simulink model "chap04"  (R2021a)
settings: Solver=FixedStepDiscrete  StartTime=0.0  StopTime=30  FixedStep=0.001  RelTol=1e-3
undefined symbols (not defined in the file): DiscIntNeverNeededParam
libraries: simulink x4
(part 1 of 7)
settings Model: Creator=陈天兴  LastModifiedBy=陈天兴

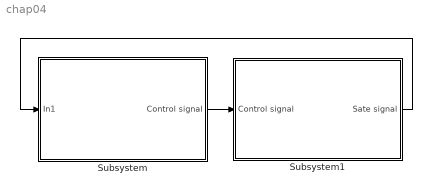
== system chap04 ==
  Subsystem : Subsystem
  Subsystem1 : Subsystem
  wires:
  Subsystem/1(Control signal) -> Subsystem1/1(Control signal)
  Subsystem1/1(Sate signal) -> Subsystem/1(In1)

== system chap04/Subsystem ==
  In1 : Inport
  Bus Creator : BusCreator  Inputs=6
  Bus Creator1 : BusCreator  Inputs=6
  Bus Creator2 : BusCreator  Inputs=3
  Subsystem : Subsystem
  Subsystem1 : Subsystem
  Subsystem10 : Subsystem
  Subsystem11 : Subsystem
  Subsystem13 : Subsystem
  Subsystem2 : Subsystem
  Subsystem3 : Subsystem
  Subsystem4 : Subsystem
  Subsystem5 : Subsystem
  Subsystem6 : Subsystem
  Subsystem7 : Subsystem
  Subsystem9 : Subsystem
  Control signal : Outport
  wires:
  Bus Creator2/1 -> Subsystem13/1(In19), Subsystem9/1(In19), Subsystem7/1(In19), Subsystem11/1(In19), Subsystem10/1(In19), Subsystem6/1(In19), Subsystem/1(In19), Subsystem2/1(In19), Subsystem5/1(In19), Subsystem4/1(In19), Subsystem1/1(In19), Subsystem3/1(In19)
  Subsystem5/1(u3) -> Bus Creator/3
  Subsystem3/1(u4) -> Bus Creator/4
  Subsystem1/1(u5) -> Bus Creator/5
  Subsystem/1(u1) -> Bus Creator/1
  Subsystem2/1(u2) -> Bus Creator/2
  Subsystem4/1(u6) -> Bus Creator/6
  Bus Creator/1 -> [control], Control signal/1
  Subsystem10/1(u4) -> Bus Creator1/4
  In1/1 -> Bus Creator2/2  "state(t)"
  Bus Creator1/1 -> Bus Creator2/1  "state(tk)"
  Subsystem6/1(u1) -> Bus Creator1/1
  Subsystem13/1(u2) -> Bus Creator1/2
  Subsystem9/1(u3) -> Bus Creator1/3
  Subsystem7/1(u5) -> Bus Creator1/5
  Subsystem11/1(u6) -> Bus Creator1/6
  [control] -> Bus Creator2/3  "control"

== system chap04/Subsystem1 ==
  Control signal : Inport
  Bus Creator : BusCreator  Inputs=7
  Bus Creator1 : BusCreator  Inputs=6
  Bus Selector : BusSelector  OutputSignals=node1.ux,node1.uy,node1.uz
  Bus Selector1 : BusSelector  OutputSignals=node2.ux,node2.uy,node2.uz
  Bus Selector2 : BusSelector  OutputSignals=node3.ux,node3.uy,node3.uz
  Bus Selector3 : BusSelector  OutputSignals=node4.ux,node4.uy,node4.uz
  Bus Selector4 : BusSelector  OutputSignals=node5.ux,node5.uy,node5.uz
  Bus Selector5 : BusSelector  OutputSignals=node6.ux,node6.uy,node6.uz
  Constant2 : Constant
  Scope : Scope  NumInputPorts=3
  Subsystem : Subsystem
  Subsystem1 : Subsystem
  Subsystem2 : Subsystem
  Subsystem3 : Subsystem
  Subsystem4 : Subsystem
  Subsystem5 : Subsystem
  Subsystem6 : Subsystem
  Subsystem7 : Subsystem
  Sate signal : Outport
  wires:
  Bus Creator/1 -> Sate signal/1
  Control signal/1 -> Bus Selector/1, Bus Selector1/1, Bus Selector5/1, Bus Selector4/1, Bus Selector3/1, Bus Selector2/1
  Bus Selector/1 -> Subsystem/4(ut1x)  "<ux>"
  Bus Selector/2 -> Subsystem/5(ut1y)  "<uy>"
  Bus Selector/3 -> Subsystem/6(ut1z)  "<uz>"
  Bus Selector1/1 -> Subsystem1/4(ut2x)  "<ux>"
  Bus Selector1/2 -> Subsystem1/5(ut2y)  "<uy>"
  Bus Selector1/3 -> Subsystem1/6(ut2z)  "<uz>"
  Bus Selector2/1 -> Subsystem2/4(ut3x)  "<ux>"
  Bus Selector2/2 -> Subsystem2/5(ut3y)  "<uy>"
  Bus Selector2/3 -> Subsystem2/6(ut3z)  "<uz>"
  Bus Selector3/1 -> Subsystem3/4(ut4x)  "<ux>"
  Bus Selector3/2 -> Subsystem3/5(ut4y)  "<uy>"
  Bus Selector3/3 -> Subsystem3/6(ut4z)  "<uz>"
  Bus Selector4/1 -> Subsystem4/4(ut5x)  "<ux>"
  Bus Selector4/2 -> Subsystem4/5(ut5y)  "<uy>"
  Bus Selector4/3 -> Subsystem4/6(ut5z)  "<uz>"
  Bus Selector5/1 -> Subsystem5/4(ut6x)  "<ux>"
  Bus Selector5/2 -> Subsystem5/5(ut6y)  "<uy>"
  Bus Selector5/3 -> Subsystem5/6(ut6z)  "<uz>"
  Subsystem5/1(node6) -> Bus Creator/7
  Subsystem4/1(node5) -> Bus Creator/6
  Subsystem3/1(node4) -> Bus Creator/5
  Subsystem2/1(node3) -> Bus Creator/4
  Subsystem1/1(node2) -> Bus Creator/3
  Subsystem/1(node1) -> Bus Creator/2
  Subsystem6/5(vy) -> Bus Creator1/5  "vy"
  Subsystem6/2(xy) -> Bus Creator1/2  "xy"
  Subsystem6/3(xz) -> Bus Creator1/3  "xz"
  Subsystem6/4(vx) -> Bus Creator1/4  "vx"
  Subsystem6/6(vz) -> Bus Creator1/6  "vz"
  Bus Creator1/1 -> Bus Creator/1  "node0"
  Subsystem6/1(xx) -> Bus Creator1/1  "xx"
  Subsystem7/2(dy) -> Subsystem/2(dy), Subsystem5/2(dy), Subsystem4/2(dy), Subsystem3/2(dy), Subsystem2/2(dy), Subsystem1/2(dy), Scope/2  "dy"
  Subsystem7/3(dz) -> Subsystem5/3(dz), Subsystem4/3(dz), Subsystem3/3(dz), Subsystem2/3(dz), Subsystem1/3(dz), Subsystem/3(dz), Scope/3  "dz"
  Subsystem7/1(dx) -> Subsystem3/1(dx), Subsystem5/1(dx), Subsystem4/1(dx), Subsystem2/1(dx), Subsystem1/1(dx), Subsystem/1(dx), Scope/1  "dx"
  Constant2/1 -> Subsystem7/1(switch)

== system chap04/Subsystem/Subsystem ==
  In19 : Inport
  Bus Creator : BusCreator  Inputs=3
  Bus Selector : BusSelector  OutputSignals=state(tk).node1.xx,state(tk).node2.xx,state(tk).node3.xx,state(tk).node6.xx,state(tk).node1.vx,state(tk).node2.vx,state(tk).node3.vx,state(tk).node6.vx
  Bus Selector1 : BusSelector  OutputSignals=state(tk).node1.xy,state(tk).node2.xy,state(tk).node3.xy,state(tk).node6.xy,state(tk).node1.vy,state(tk).node2.vy,state(tk).node3.vy,state(tk).node6.vy
  Bus Selector2 : BusSelector  OutputSignals=state(tk).node1.xz,state(tk).node2.xz,state(tk).node3.xz,state(tk).node6.xz,state(tk).node1.vz,state(tk).node2.vz,state(tk).node3.vz,state(tk).node6.vz
  Bus Selector3 : BusSelector  OutputSignals=state(t).node1.vx
  Bus Selector4 : BusSelector  OutputSignals=state(t).node1.vy
  Bus Selector5 : BusSelector  OutputSignals=state(t).node1.vz
  Bus Selector6 : BusSelector  OutputSignals=state(t).node1.vx,state(t).node1.vy,state(t).node1.vz
  Bus Selector7 : BusSelector  OutputSignals=state(t).node1.vx,state(t).node1.vy,state(t).node1.vz
  Bus Selector8 : BusSelector  OutputSignals=control.node1.ux,control.node1.uy,control.node1.uz
  Subsystem1 : Subsystem
  Subsystem10 : Subsystem
  Subsystem12 : Subsystem
  Subsystem2 : Subsystem
  Subsystem3 : Subsystem
  Subsystem4 : Subsystem
      settings: PortSchema="{\"entries\":[{\"content\":{\"sides\":[{\"content\":{\"connectorIds\":[\"In1\",\"In2\",\"In3\"]},\"type\":\"ConnectorPlacement.EquallySpacedRectSide\",\"uuid\":\"3c32f130-2df4-4697-80e9-267a8217898e\"},{\"content\":{\"connectorIds\":[\"Out1\"],\"side\":\"RIGHT\"},\"type\":\"ConnectorPlacement.EquallySpacedRectSide\",\"uuid\":\"840675a7-4714-440f-a6ce-75eff1b2763f\"},{\"content\":{\"connectorIds\":[],\"side\":\"TOP\"},\"type\":\"ConnectorPlacement.EquallySpacedRectSide\",\"uuid\":\"5c23af56-4ec3-4a39-a531-12998a0be3c8\"},{\"content\":{\"connectorIds\":[\"Out2\"],\"side\":\"BOTTOM\"},\"type\":\"ConnectorPlacement.EquallySpacedRectSide\",\"uuid\":\"31d953fb-65a0-42e9-a844-060de010f298\"}]},\"type\":\"ConnectorPlacement.EquallySpacedConnector\",\"uuid\":\"61b27aa3-5880-401e-bae3-4611093a191a\"}],\"packageUris\":[\"http://schema.mathworks.com/mf0/Connector/R2020b\"],\"version\":\"1.0\"}"
  Subsystem6 : Subsystem
  Subsystem7 : Subsystem
      settings: PortSchema="{\"entries\":[{\"content\":{\"sides\":[{\"content\":{\"connectorIds\":[\"In1\",\"In2\",\"In3\"]},\"type\":\"ConnectorPlacement.EquallySpacedRectSide\",\"uuid\":\"3c32f130-2df4-4697-80e9-267a8217898e\"},{\"content\":{\"connectorIds\":[\"Out1\"],\"side\":\"RIGHT\"},\"type\":\"ConnectorPlacement.EquallySpacedRectSide\",\"uuid\":\"840675a7-4714-440f-a6ce-75eff1b2763f\"},{\"content\":{\"connectorIds\":[],\"side\":\"TOP\"},\"type\":\"ConnectorPlacement.EquallySpacedRectSide\",\"uuid\":\"5c23af56-4ec3-4a39-a531-12998a0be3c8\"},{\"content\":{\"connectorIds\":[\"Out2\"],\"side\":\"BOTTOM\"},\"type\":\"ConnectorPlacement.EquallySpacedRectSide\",\"uuid\":\"31d953fb-65a0-42e9-a844-060de010f298\"}]},\"type\":\"ConnectorPlacement.EquallySpacedConnector\",\"uuid\":\"61b27aa3-5880-401e-bae3-4611093a191a\"}],\"packageUris\":[\"http://schema.mathworks.com/mf0/Connector/R2020b\"],\"version\":\"1.0\"}"
  Subsystem8 : Subsystem
      settings: PortSchema="{\"entries\":[{\"content\":{\"sides\":[{\"content\":{\"connectorIds\":[\"In1\",\"In2\",\"In3\"]},\"type\":\"ConnectorPlacement.EquallySpacedRectSide\",\"uuid\":\"3c32f130-2df4-4697-80e9-267a8217898e\"},{\"content\":{\"connectorIds\":[\"Out1\"],\"side\":\"RIGHT\"},\"type\":\"ConnectorPlacement.EquallySpacedRectSide\",\"uuid\":\"840675a7-4714-440f-a6ce-75eff1b2763f\"},{\"content\":{\"connectorIds\":[],\"side\":\"TOP\"},\"type\":\"ConnectorPlacement.EquallySpacedRectSide\",\"uuid\":\"5c23af56-4ec3-4a39-a531-12998a0be3c8\"},{\"content\":{\"connectorIds\":[\"Out2\"],\"side\":\"BOTTOM\"},\"type\":\"ConnectorPlacement.EquallySpacedRectSide\",\"uuid\":\"31d953fb-65a0-42e9-a844-060de010f298\"}]},\"type\":\"ConnectorPlacement.EquallySpacedConnector\",\"uuid\":\"61b27aa3-5880-401e-bae3-4611093a191a\"}],\"packageUris\":[\"http://schema.mathworks.com/mf0/Connector/R2020b\"],\"version\":\"1.0\"}"
  u1 : Outport
  wires:
  Subsystem2/1(utx) -> Subsystem8/2(utz)
  Subsystem6/1(utx) -> Subsystem4/2(utx)
  Subsystem1/1(utx) -> Subsystem7/2(uty)
  Bus Creator/1 -> u1/1  "node1"
  In19/1 -> [state], Bus Selector2/1, Bus Selector/1, Bus Selector1/1
  Bus Selector/1 -> Subsystem6/1(xx1)  "<xx>"
  Bus Selector/2 -> Subsystem6/2(xx2)  "<xx>"
  Bus Selector/3 -> Subsystem6/3(xx3)  "<xx>"
  Bus Selector/4 -> Subsystem6/4(xx6)  "<xx>"
  Bus Selector/5 -> Subsystem6/5(vx1)  "<vx>"
  Bus Selector/6 -> Subsystem6/6(vx2)  "<vx>"
  Bus Selector/7 -> Subsystem6/7(vx3)  "<vx>"
  Bus Selector/8 -> Subsystem6/8(vx6)  "<vx>"
  Bus Selector1/1 -> Subsystem1/1(xy1)  "<xy>"
  Bus Selector1/2 -> Subsystem1/2(xy2)  "<xy>"
  Bus Selector1/3 -> Subsystem1/3(xy3)  "<xy>"
  Bus Selector1/4 -> Subsystem1/4(xy6)  "<xy>"
  Bus Selector1/5 -> Subsystem1/5(vy1)  "<vy>"
  Bus Selector1/6 -> Subsystem1/6(vy2)  "<vy>"
  Bus Selector1/7 -> Subsystem1/7(vy3)  "<vy>"
  Bus Selector1/8 -> Subsystem1/8(vy6)  "<vy>"
  Bus Selector2/1 -> Subsystem2/1(xz1)  "<xz>"
  Bus Selector2/2 -> Subsystem2/2(xx2)  "<xz>"
  Bus Selector2/3 -> Subsystem2/3(xz3)  "<xz>"
  Bus Selector2/4 -> Subsystem2/4(xz6)  "<xz>"
  Bus Selector2/5 -> Subsystem2/5(vz1)  "<vz>"
  Bus Selector2/6 -> Subsystem2/6(vz2)  "<vz>"
  Bus Selector2/7 -> Subsystem2/7(vz3)  "<vz>"
  Bus Selector2/8 -> Subsystem2/8(vz6)  "<vz>"
  [state] -> Bus Selector3/1
  Bus Selector3/1 -> Subsystem4/1(vx1)  "<vx>"
  Bus Selector4/1 -> Subsystem7/1(vy1)  "<vy>"
  [state] -> Bus Selector4/1
  [state] -> Bus Selector5/1
  Bus Selector5/1 -> Subsystem8/1(vz1)  "<vz>"
  [state] -> Bus Selector6/1
  Bus Selector6/2 -> Subsystem12/5(vy)  "<vy>"
  Bus Selector6/1 -> Subsystem12/4(vx)  "<vx>"
  Bus Selector6/3 -> Subsystem12/6(vz)  "<vz>"
  Subsystem12/1(" gain") -> [gain]
  [gain] -> Subsystem8/3(gain)
  [gain] -> Subsystem7/3(gain)
  [gain] -> Subsystem4/3(gain)
  Subsystem4/2(Sx) -> [Sx]
  Subsystem7/2(Sy) -> [Sy]
  Subsystem8/2(Sz) -> [Sz]
  [Sx] -> Subsystem12/1(Sx)
  [Sy] -> Subsystem12/2(Sy)
  [Sz] -> Subsystem12/3(Sz)
  Subsystem10/1(ux) -> Bus Creator/1  "ux"
  Subsystem10/2(uy) -> Bus Creator/2  "uy"
  Subsystem10/3(uz) -> Bus Creator/3  "uz"
  Subsystem4/1(ux) -> Subsystem3/1(utx)
  Subsystem7/1(ux) -> Subsystem3/5(uty)
  Subsystem8/1(ux) -> Subsystem3/9(utz)
  [state] -> Bus Selector7/1
  Bus Selector7/1 -> Subsystem3/2(vx)  "<vx>"
  Bus Selector7/2 -> Subsystem3/3(vy)  "<vy>"
  Bus Selector7/3 -> Subsystem3/4(vz)  "<vz>"
  [state] -> Bus Selector8/1
  Bus Selector8/1 -> Subsystem3/6(ux)  "<ux>"
  Bus Selector8/2 -> Subsystem3/7(uy)  "<uy>"
  Bus Selector8/3 -> Subsystem3/8(uz)  "<uz>"
  Subsystem3/1(udtx) -> Subsystem10/1(utx)
  Subsystem3/2(udty) -> Subsystem10/2(uty)
  Subsystem3/3(udtz) -> Subsystem10/3(utz)

== system chap04/Subsystem/Subsystem1 ==
  In19 : Inport
  Bus Creator : BusCreator  Inputs=3
  Bus Selector : BusSelector  OutputSignals=state(tk).node5.xx,state(tk).node5.xx0,state(tk).node3.xx,state(tk).node4.xx,state(tk).node5.vx,state(tk).node5.vx0,state(tk).node3.vx,state(tk).node4.vx
  Bus Selector1 : BusSelector  OutputSignals=state(tk).node5.xy,state(tk).node5.xy0,state(tk).node3.xy,state(tk).node4.xy,state(tk).node5.vy,state(tk).node5.vy0,state(tk).node3.vy,state(tk).node4.vy
  Bus Selector2 : BusSelector  OutputSignals=state(tk).node5.xz,state(tk).node5.xz0,state(tk).node3.xz,state(tk).node4.xz,state(tk).node5.vz,state(tk).node5.vz0,state(tk).node3.vz,state(tk).node4.vz
  Bus Selector3 : BusSelector  OutputSignals=state(t).node5.vx,state(t).node0.vx
  Bus Selector4 : BusSelector  OutputSignals=state(t).node5.vy,state(t).node0.vx
  Bus Selector5 : BusSelector  OutputSignals=state(t).node5.vz,state(t).node0.vz
  Bus Selector6 : BusSelector  OutputSignals=state(t).node5.vx,state(t).node5.vy,state(t).node5.vz
  Bus Selector7 : BusSelector  OutputSignals=state(t).node5.vx,state(t).node5.vy,state(t).node5.vz
  Bus Selector8 : BusSelector  OutputSignals=control.node5.ux,control.node5.uy,control.node5.uz
  Subsystem1 : Subsystem
  Subsystem10 : Subsystem
  Subsystem12 : Subsystem
  Subsystem2 : Subsystem
  Subsystem3 : Subsystem
  Subsystem4 : Subsystem
      settings: PortSchema="{\"entries\":[{\"content\":{\"sides\":[{\"content\":{\"connectorIds\":[\"In1\",\"In2\",\"In3\",\"In4\"]},\"type\":\"ConnectorPlacement.EquallySpacedRectSide\",\"uuid\":\"3c32f130-2df4-4697-80e9-267a8217898e\"},{\"content\":{\"connectorIds\":[\"Out1\"],\"side\":\"RIGHT\"},\"type\":\"ConnectorPlacement.EquallySpacedRectSide\",\"uuid\":\"840675a7-4714-440f-a6ce-75eff1b2763f\"},{\"content\":{\"connectorIds\":[],\"side\":\"TOP\"},\"type\":\"ConnectorPlacement.EquallySpacedRectSide\",\"uuid\":\"5c23af56-4ec3-4a39-a531-12998a0be3c8\"},{\"content\":{\"connectorIds\":[\"Out2\"],\"side\":\"BOTTOM\"},\"type\":\"ConnectorPlacement.EquallySpacedRectSide\",\"uuid\":\"31d953fb-65a0-42e9-a844-060de010f298\"}]},\"type\":\"ConnectorPlacement.EquallySpacedConnector\",\"uuid\":\"61b27aa3-5880-401e-bae3-4611093a191a\"}],\"packageUris\":[\"http://schema.mathworks.com/mf0/Connector/R2020b\"],\"version\":\"1.0\"}"
  Subsystem6 : Subsystem
  Subsystem7 : Subsystem
      settings: PortSchema="{\"entries\":[{\"content\":{\"sides\":[{\"content\":{\"connectorIds\":[\"In1\",\"In2\",\"In3\",\"In4\"]},\"type\":\"ConnectorPlacement.EquallySpacedRectSide\",\"uuid\":\"3c32f130-2df4-4697-80e9-267a8217898e\"},{\"content\":{\"connectorIds\":[\"Out1\"],\"side\":\"RIGHT\"},\"type\":\"ConnectorPlacement.EquallySpacedRectSide\",\"uuid\":\"840675a7-4714-440f-a6ce-75eff1b2763f\"},{\"content\":{\"connectorIds\":[],\"side\":\"TOP\"},\"type\":\"ConnectorPlacement.EquallySpacedRectSide\",\"uuid\":\"5c23af56-4ec3-4a39-a531-12998a0be3c8\"},{\"content\":{\"connectorIds\":[\"Out2\"],\"side\":\"BOTTOM\"},\"type\":\"ConnectorPlacement.EquallySpacedRectSide\",\"uuid\":\"31d953fb-65a0-42e9-a844-060de010f298\"}]},\"type\":\"ConnectorPlacement.EquallySpacedConnector\",\"uuid\":\"61b27aa3-5880-401e-bae3-4611093a191a\"}],\"packageUris\":[\"http://schema.mathworks.com/mf0/Connector/R2020b\"],\"version\":\"1.0\"}"
  Subsystem8 : Subsystem
      settings: PortSchema="{\"entries\":[{\"content\":{\"sides\":[{\"content\":{\"connectorIds\":[\"In1\",\"In2\",\"In3\",\"In4\"]},\"type\":\"ConnectorPlacement.EquallySpacedRectSide\",\"uuid\":\"3c32f130-2df4-4697-80e9-267a8217898e\"},{\"content\":{\"connectorIds\":[\"Out1\"],\"side\":\"RIGHT\"},\"type\":\"ConnectorPlacement.EquallySpacedRectSide\",\"uuid\":\"840675a7-4714-440f-a6ce-75eff1b2763f\"},{\"content\":{\"connectorIds\":[],\"side\":\"TOP\"},\"type\":\"ConnectorPlacement.EquallySpacedRectSide\",\"uuid\":\"5c23af56-4ec3-4a39-a531-12998a0be3c8\"},{\"content\":{\"connectorIds\":[\"Out2\"],\"side\":\"BOTTOM\"},\"type\":\"ConnectorPlacement.EquallySpacedRectSide\",\"uuid\":\"31d953fb-65a0-42e9-a844-060de010f298\"}]},\"type\":\"ConnectorPlacement.EquallySpacedConnector\",\"uuid\":\"61b27aa3-5880-401e-bae3-4611093a191a\"}],\"packageUris\":[\"http://schema.mathworks.com/mf0/Connector/R2020b\"],\"version\":\"1.0\"}"
  u5 : Outport
  wires:
  Bus Creator/1 -> u5/1  "node5"
  Bus Selector/5 -> Subsystem6/5(vx5)  "<vx>"
  Bus Selector/1 -> Subsystem6/1(xx5)  "<xx>"
  Bus Selector/3 -> Subsystem6/3(xx3)  "<xx>"
  Bus Selector/8 -> Subsystem6/8(vx4)  "<vx>"
  Bus Selector/7 -> Subsystem6/7(vx3)  "<vx>"
  Bus Selector/4 -> Subsystem6/4(xx4)  "<xx>"
  Bus Selector6/3 -> Subsystem12/6(vz)  "<vz>"
  Bus Selector6/1 -> Subsystem12/4(vx)  "<vx>"
  [Sx] -> Subsystem12/1(Sx)
  [Sz] -> Subsystem12/3(Sz)
  Subsystem12/1(" gain") -> [gain]
  In19/1 -> [state], Bus Selector2/1, Bus Selector/1, Bus Selector1/1
  [state] -> Bus Selector6/1
  [Sy] -> Subsystem12/2(Sy)
  Bus Selector6/2 -> Subsystem12/5(vy)  "<vy>"
  Subsystem10/3(uz) -> Bus Creator/3  "uz"
  Subsystem10/2(uy) -> Bus Creator/2  "uy"
  Subsystem10/1(ux) -> Bus Creator/1  "ux"
  [state] -> Bus Selector7/1
  Bus Selector8/1 -> Subsystem3/6(ux)  "<ux>"
  Bus Selector7/2 -> Subsystem3/3(vy)  "<vy>"
  Bus Selector8/2 -> Subsystem3/7(uy)  "<uy>"
  [state] -> Bus Selector8/1
  Bus Selector7/1 -> Subsystem3/2(vx)  "<vx>"
  Bus Selector7/3 -> Subsystem3/4(vz)  "<vz>"
  Bus Selector8/3 -> Subsystem3/8(uz)  "<uz>"
  Subsystem3/1(udtx) -> Subsystem10/1(utx)
  Subsystem3/2(udty) -> Subsystem10/2(uty)
  Subsystem3/3(udtz) -> Subsystem10/3(utz)
  Bus Selector/2 -> Subsystem6/2(xx0)  "<xx0>"
  Bus Selector/6 -> Subsystem6/6(vx0)  "<vx0>"
  Bus Selector1/1 -> Subsystem1/1(xy5)  "<xy>"
  Bus Selector1/2 -> Subsystem1/2(xy0)  "<xy0>"
  Bus Selector1/3 -> Subsystem1/3(xy3)  "<xy>"
  Bus Selector1/4 -> Subsystem1/4(xy4)  "<xy>"
  Bus Selector1/5 -> Subsystem1/5(vy5)  "<vy>"
  Bus Selector1/6 -> Subsystem1/6(vy0)  "<vy0>"
  Bus Selector1/7 -> Subsystem1/7(vy3)  "<vy>"
  Bus Selector1/8 -> Subsystem1/8(vy4)  "<vy>"
  Bus Selector2/1 -> Subsystem2/1(xz5)  "<xz>"
  Bus Selector2/2 -> Subsystem2/2(xz0)  "<xz0>"
  Bus Selector2/3 -> Subsystem2/3(xz3)  "<xz>"
  Bus Selector2/4 -> Subsystem2/4(xz4)  "<xz>"
  Bus Selector2/5 -> Subsystem2/5(vz5)  "<vz>"
  Bus Selector2/6 -> Subsystem2/6(vz0)  "<vz0>"
  Bus Selector2/7 -> Subsystem2/7(vz3)  "<vz>"
  Bus Selector2/8 -> Subsystem2/8(vz4)  "<vz>"
  [gain] -> Subsystem8/4(gain)
  Subsystem7/1(ux) -> Subsystem3/5(uty)
  Subsystem2/1(utz) -> Subsystem8/3(utz)
  Subsystem1/1(uty) -> Subsystem7/3(uty)
  [state] -> Bus Selector3/1
  Subsystem4/1(ux) -> Subsystem3/1(utx)
  Bus Selector3/2 -> Subsystem4/2(vx0)  "<vx>"
  Bus Selector3/1 -> Subsystem4/1(vx5)  "<vx>"
  Subsystem8/1(ux) -> Subsystem3/9(utz)
  Bus Selector5/1 -> Subsystem8/1(vz5)  "<vz>"
  [state] -> Bus Selector4/1
  Subsystem6/1(utx) -> Subsystem4/3(utx)
  [state] -> Bus Selector5/1
  Bus Selector4/1 -> Subsystem7/1(vy5)  "<vy>"
  Bus Selector4/2 -> Subsystem7/2(vy0)  "<vx>"
  Bus Selector5/2 -> Subsystem8/2(vz0)  "<vz>"
  [gain] -> Subsystem4/4(gain)
  Subsystem4/2(Sx) -> [Sx]
  Subsystem7/2(Sy) -> [Sy]
  Subsystem8/2(Sz) -> [Sz]
  [gain] -> Subsystem7/4(gain)

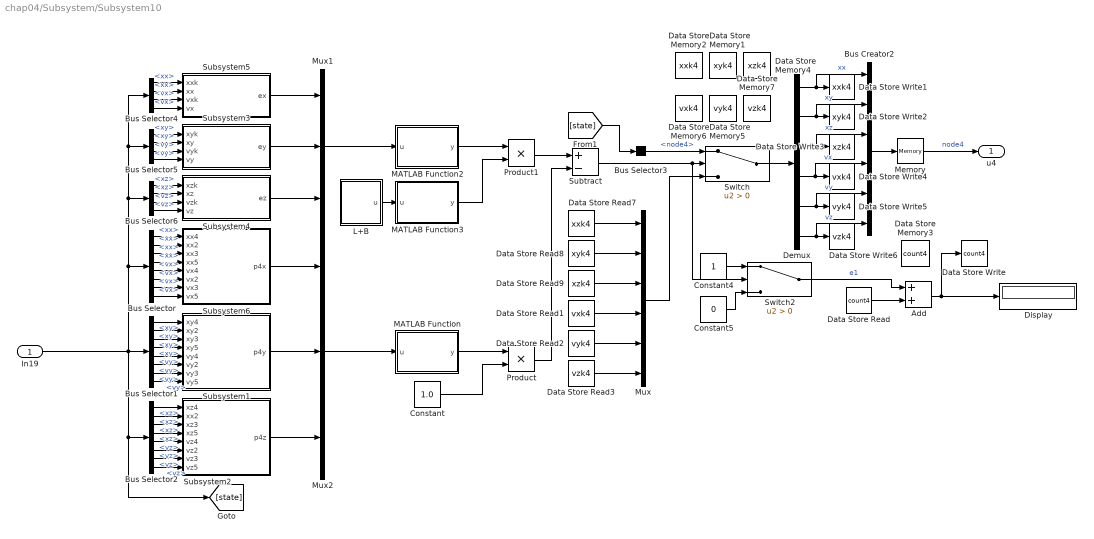
== system chap04/Subsystem/Subsystem10 ==
  In19 : Inport
  Add : Sum
  Bus Creator2 : BusCreator  Inputs=6
  Bus Selector : BusSelector  OutputSignals=state(tk).node4.xx,state(tk).node2.xx,state(tk).node3.xx,state(tk).node5.xx,state(tk).node4.vx,state(tk).node2.vx,state(tk).node3.vx,state(tk).node5.vx
  Bus Selector1 : BusSelector  OutputSignals=state(tk).node4.xy,state(tk).node2.xy,state(tk).node3.xy,state(tk).node5.xy,state(tk).node4.vy,state(tk).node2.vy,state(tk).node3.vy,state(tk).node5.vy
  Bus Selector2 : BusSelector  OutputSignals=state(tk).node4.xz,state(tk).node2.xz,state(tk).node3.xz,state(tk).node5.xz,state(tk).node4.vz,state(tk).node2.vz,state(tk).node3.vz,state(tk).node5.vz
  Bus Selector3 : BusSelector  OutputSignals=state(t).node4
  Bus Selector4 : BusSelector  OutputSignals=state(tk).node4.xx,state(t).node4.xx,state(tk).node4.vx,state(t).node4.vx
  Bus Selector5 : BusSelector  OutputSignals=state(tk).node4.xy,state(t).node4.xy,state(tk).node4.vy,state(t).node4.vy
  Bus Selector6 : BusSelector  OutputSignals=state(tk).node4.xz,state(t).node4.xz,state(tk).node4.vz,state(t).node4.vz
  Constant : Constant  Value=1.0
  Constant4 : Constant
  Constant5 : Constant  Value=0
  Data Store Memory1 : DataStoreMemory  DataStoreName=xyk4  ReadBeforeWriteMsg=warning  WriteAfterWriteMsg=warning  WriteAfterReadMsg=warning  ShowAdditionalParam=off
  Data Store Memory2 : DataStoreMemory  DataStoreName=xxk4  ReadBeforeWriteMsg=warning  WriteAfterWriteMsg=warning  WriteAfterReadMsg=warning  ShowAdditionalParam=off
  Data Store Memory3 : DataStoreMemory  DataStoreName=count4  ReadBeforeWriteMsg=warning  WriteAfterWriteMsg=warning  WriteAfterReadMsg=warning  ShowAdditionalParam=off
  Data Store Memory4 : DataStoreMemory  DataStoreName=xzk4  ReadBeforeWriteMsg=warning  WriteAfterWriteMsg=warning  WriteAfterReadMsg=warning  ShowAdditionalParam=off
  Data Store Memory5 : DataStoreMemory  DataStoreName=vyk4  ReadBeforeWriteMsg=warning  WriteAfterWriteMsg=warning  WriteAfterReadMsg=warning  ShowAdditionalParam=off
  Data Store Memory6 : DataStoreMemory  DataStoreName=vxk4  ReadBeforeWriteMsg=warning  WriteAfterWriteMsg=warning  WriteAfterReadMsg=warning  ShowAdditionalParam=off
  Data Store Memory7 : DataStoreMemory  DataStoreName=vzk4  ReadBeforeWriteMsg=warning  WriteAfterWriteMsg=warning  WriteAfterReadMsg=warning  ShowAdditionalParam=off
  Data Store Read : DataStoreRead  DataStoreName=count4  IndexOptions=Index vector (dialog)  Indices=1  OutputSizes=1
  Data Store Read1 : DataStoreRead  DataStoreName=vxk4  IndexOptions=Index vector (dialog)  Indices=1  OutputSizes=1
  Data Store Read2 : DataStoreRead  DataStoreName=vyk4  IndexOptions=Index vector (dialog)  Indices=1  OutputSizes=1
  Data Store Read3 : DataStoreRead  DataStoreName=vzk4  IndexOptions=Index vector (dialog)  Indices=1  OutputSizes=1
  Data Store Read7 : DataStoreRead  DataStoreName=xxk4  IndexOptions=Index vector (dialog)  Indices=1  OutputSizes=1
  Data Store Read8 : DataStoreRead  DataStoreName=xyk4  IndexOptions=Index vector (dialog)  Indices=1  OutputSizes=1
  Data Store Read9 : DataStoreRead  DataStoreName=xzk4  IndexOptions=Index vector (dialog)  Indices=1  OutputSizes=1
  Data Store Write : DataStoreWrite  DataStoreName=count4  IndexOptions=Index vector (dialog)  Indices=1  OutputSizes=1
  Data Store Write1 : DataStoreWrite  DataStoreName=xxk4  IndexOptions=Index vector (dialog)  Indices=1  OutputSizes=1
  Data Store Write2 : DataStoreWrite  DataStoreName=xyk4  IndexOptions=Index vector (dialog)  Indices=1  OutputSizes=1
  Data Store Write3 : DataStoreWrite  DataStoreName=xzk4  IndexOptions=Index vector (dialog)  Indices=1  OutputSizes=1
  Data Store Write4 : DataStoreWrite  DataStoreName=vxk4  IndexOptions=Index vector (dialog)  Indices=1  OutputSizes=1
  Data Store Write5 : DataStoreWrite  DataStoreName=vyk4  IndexOptions=Index vector (dialog)  Indices=1  OutputSizes=1
  Data Store Write6 : DataStoreWrite  DataStoreName=vzk4  IndexOptions=Index vector (dialog)  Indices=1  OutputSizes=1
  Demux : Demux  Outputs=6
  Display : Display
  L+B : Subsystem
  MATLAB Function : MATLAB Function  TreatAsAtomicUnit=on
  MATLAB Function2 : MATLAB Function  TreatAsAtomicUnit=on
  MATLAB Function3 : MATLAB Function  TreatAsAtomicUnit=on
  Memory : Memory
  Mux : Mux  Inputs=6
  Mux1 : Mux  Inputs=3
  Mux2 : Mux  Inputs=3
  Product : Product
  Product1 : Product
  Subsystem1 : Subsystem
  Subsystem2 : Subsystem
  Subsystem3 : Subsystem
  Subsystem4 : Subsystem
  Subsystem5 : Subsystem
  Subsystem6 : Subsystem
  Subtract : Sum  Inputs=+-
  Switch : Switch  Criteria=u2 > Threshold
  Switch2 : Switch  Criteria=u2 > Threshold
  u4 : Outport
  wires:
  Subsystem2/1(p4z) -> Mux2/3
  Subsystem6/1(p4x) -> Mux2/1
  Subsystem1/1(p4y) -> Mux2/2
  Bus Selector/1 -> Subsystem6/1(xx4)  "<xx>"
  Bus Selector/2 -> Subsystem6/2(xx2)  "<xx>"
  Bus Selector/3 -> Subsystem6/3(xx3)  "<xx>"
  Bus Selector/4 -> Subsystem6/4(xx5)  "<xx>"
  Bus Selector/5 -> Subsystem6/5(vx4)  "<vx>"
  Bus Selector/6 -> Subsystem6/6(vx2)  "<vx>"
  Bus Selector/7 -> Subsystem6/7(vx3)  "<vx>"
  Bus Selector/8 -> Subsystem6/8(vx5)  "<vx>"
  Bus Selector1/1 -> Subsystem1/1(xy4)  "<xy>"
  Bus Selector1/2 -> Subsystem1/2(xy2)  "<xy>"
  Bus Selector1/3 -> Subsystem1/3(xy3)  "<xy>"
  Bus Selector1/4 -> Subsystem1/4(xy5)  "<xy>"
  Bus Selector1/5 -> Subsystem1/5(vy4)  "<vy>"
  Bus Selector1/6 -> Subsystem1/6(vy2)  "<vy>"
  Bus Selector1/7 -> Subsystem1/7(vy3)  "<vy>"
  Bus Selector1/8 -> Subsystem1/8(vy5)  "<vy>"
  Bus Selector2/1 -> Subsystem2/1(xz4)  "<xz>"
  Bus Selector2/2 -> Subsystem2/2(xx2)  "<xz>"
  Bus Selector2/3 -> Subsystem2/3(xz3)  "<xz>"
  Bus Selector2/4 -> Subsystem2/4(xz5)  "<xz>"
  Bus Selector2/5 -> Subsystem2/5(vz4)  "<vz>"
  Bus Selector2/6 -> Subsystem2/6(vz2)  "<vz>"
  Bus Selector2/7 -> Subsystem2/7(vz3)  "<vz>"
  Bus Selector2/8 -> Subsystem2/8(vz5)  "<vz>"
  Data Store Read3/1 -> Mux/6
  Switch/1 -> Demux/1
  Demux/2 -> Bus Creator2/2, Data Store Write2/1  "xy"
  Bus Selector3/1 -> Switch/1  "<node4>"
  Demux/1 -> Bus Creator2/1, Data Store Write1/1  "xx"
  Switch2/1 -> Add/1  "e1"
  Demux/6 -> Bus Creator2/6, Data Store Write6/1  "vz"
  Demux/3 -> Bus Creator2/3, Data Store Write3/1  "xz"
  Data Store Read7/1 -> Mux/1
  Constant4/1 -> Switch2/1
  Mux/1 -> Switch/3
  Data Store Read9/1 -> Mux/3
  Add/1 -> Data Store Write/1, Display/1
  Demux/4 -> Bus Creator2/4, Data Store Write4/1  "vx"
  Bus Creator2/1 -> Memory/1
  Data Store Read2/1 -> Mux/5
  Data Store Read1/1 -> Mux/4
  Product/1 -> Subtract/2
  Data Store Read8/1 -> Mux/2
  [state] -> Bus Selector3/1
  MATLAB Function3/1(y) -> Product1/2
  Mux1/1 -> MATLAB Function2/1(u)
  Constant5/1 -> Switch2/3
  Constant/1 -> Product/2
  MATLAB Function2/1(y) -> Product1/1
  L+B/1(u) -> MATLAB Function3/1(u)
  Subsystem4/1(ez) -> Mux1/3
  Subsystem5/1(ex) -> Mux1/1
  Subsystem3/1(ey) -> Mux1/2
  Demux/5 -> Bus Creator2/5, Data Store Write5/1  "vy"
  Product1/1 -> Subtract/1
  Data Store Read/1 -> Add/2
  MATLAB Function/1(y) -> Product/1
  Mux2/1 -> MATLAB Function/1(u)
  Bus Selector5/3 -> Subsystem3/3(vyk)  "<vy>"
  In19/1 -> [state], Bus Selector2/1, Bus Selector1/1, Bus Selector/1, Bus Selector6/1, Bus Selector5/1, Bus Selector4/1
  Bus Selector5/2 -> Subsystem3/2(xy)  "<xy>"
  Bus Selector5/4 -> Subsystem3/4(vy)  "<vy>"
  Bus Selector5/1 -> Subsystem3/1(xyk)  "<xy>"
  Bus Selector6/2 -> Subsystem4/2(xz)  "<xz>"
  Bus Selector6/3 -> Subsystem4/3(vzk)  "<vz>"
  Bus Selector6/4 -> Subsystem4/4(vz)  "<vz>"
  Bus Selector6/1 -> Subsystem4/1(xzk)  "<xz>"
  Memory/1 -> u4/1  "node4"
  Bus Selector4/1 -> Subsystem5/1(xxk)  "<xx>"
  Bus Selector4/2 -> Subsystem5/2(xx)  "<xx>"
  Bus Selector4/3 -> Subsystem5/3(vxk)  "<vx>"
  Bus Selector4/4 -> Subsystem5/4(vx)  "<vx>"
  Subtract/1 -> Switch/2, Switch2/2

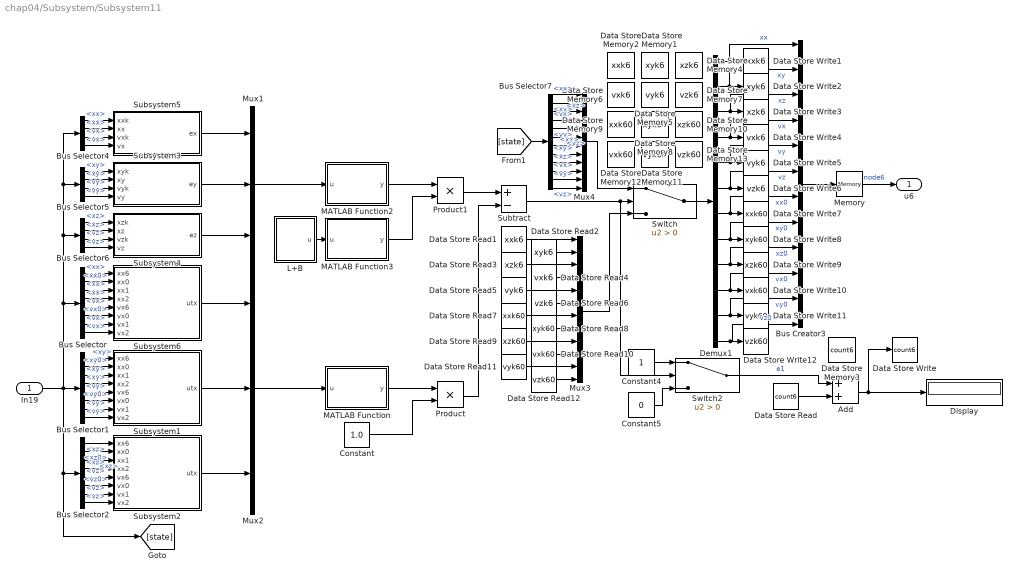
== system chap04/Subsystem/Subsystem11 ==
  In19 : Inport
  Add : Sum
  Bus Creator3 : BusCreator  Inputs=12
  Bus Selector : BusSelector  OutputSignals=state(tk).node6.xx,state(tk).node6.xx0,state(tk).node1.xx,state(tk).node2.xx,state(tk).node6.vx,state(tk).node6.vx0,state(tk).node1.vx,state(tk).node2.vx
  Bus Selector1 : BusSelector  OutputSignals=state(tk).node6.xy,state(tk).node6.xy0,state(tk).node1.xy,state(tk).node2.xy,state(tk).node6.vy,state(tk).node6.vy0,state(tk).node1.vy,state(tk).node2.vy
  Bus Selector2 : BusSelector  OutputSignals=state(tk).node6.xz,state(tk).node6.xz0,state(tk).node1.xz,state(tk).node2.xz,state(tk).node6.vz,state(tk).node6.vz0,state(tk).node1.vz,state(tk).node2.vz
  Bus Selector4 : BusSelector  OutputSignals=state(tk).node6.xx,state(t).node6.xx,state(tk).node6.vx,state(t).node6.vx
  Bus Selector5 : BusSelector  OutputSignals=state(tk).node6.xy,state(t).node6.xy,state(tk).node6.vy,state(t).node6.vy
  Bus Selector6 : BusSelector  OutputSignals=state(tk).node6.xz,state(t).node6.xz,state(tk).node6.vz,state(t).node6.vz
  Bus Selector7 : BusSelector  OutputSignals=state(t).node6.xx,state(t).node6.xy,state(t).node6.xz,state(t).node6.vx,state(t).node6.vy,state(t).node6.vz,state(t).node0.xx,state(t).node0.xy,state(t).node0.xz,state(t).node0.vx,state(t).node0.vy,state(t).node0.vz
  Constant : Constant  Value=1.0
  Constant4 : Constant
  Constant5 : Constant  Value=0
  Data Store Memory1 : DataStoreMemory  DataStoreName=xyk6  ReadBeforeWriteMsg=warning  WriteAfterWriteMsg=warning  WriteAfterReadMsg=warning  ShowAdditionalParam=off
  Data Store Memory10 : DataStoreMemory  DataStoreName=xzk60  ReadBeforeWriteMsg=warning  WriteAfterWriteMsg=warning  WriteAfterReadMsg=warning  ShowAdditionalParam=off
  Data Store Memory11 : DataStoreMemory  DataStoreName=vyk60  ReadBeforeWriteMsg=warning  WriteAfterWriteMsg=warning  WriteAfterReadMsg=warning  ShowAdditionalParam=off
  Data Store Memory12 : DataStoreMemory  DataStoreName=vxk60  ReadBeforeWriteMsg=warning  WriteAfterWriteMsg=warning  WriteAfterReadMsg=warning  ShowAdditionalParam=off
  Data Store Memory13 : DataStoreMemory  DataStoreName=vzk60  ReadBeforeWriteMsg=warning  WriteAfterWriteMsg=warning  WriteAfterReadMsg=warning  ShowAdditionalParam=off
  Data Store Memory2 : DataStoreMemory  DataStoreName=xxk6  ReadBeforeWriteMsg=warning  WriteAfterWriteMsg=warning  WriteAfterReadMsg=warning  ShowAdditionalParam=off
  Data Store Memory3 : DataStoreMemory  DataStoreName=count6  ReadBeforeWriteMsg=warning  WriteAfterWriteMsg=warning  WriteAfterReadMsg=warning  ShowAdditionalParam=off
  Data Store Memory4 : DataStoreMemory  DataStoreName=xzk6  ReadBeforeWriteMsg=warning  WriteAfterWriteMsg=warning  WriteAfterReadMsg=warning  ShowAdditionalParam=off
  Data Store Memory5 : DataStoreMemory  DataStoreName=vyk6  ReadBeforeWriteMsg=warning  WriteAfterWriteMsg=warning  WriteAfterReadMsg=warning  ShowAdditionalParam=off
  Data Store Memory6 : DataStoreMemory  DataStoreName=vxk6  ReadBeforeWriteMsg=warning  WriteAfterWriteMsg=warning  WriteAfterReadMsg=warning  ShowAdditionalParam=off
  Data Store Memory7 : DataStoreMemory  DataStoreName=vzk6  ReadBeforeWriteMsg=warning  WriteAfterWriteMsg=warning  WriteAfterReadMsg=warning  ShowAdditionalParam=off
  Data Store Memory8 : DataStoreMemory  DataStoreName=xyk60  ReadBeforeWriteMsg=warning  WriteAfterWriteMsg=warning  WriteAfterReadMsg=warning  ShowAdditionalParam=off
  Data Store Memory9 : DataStoreMemory  DataStoreName=xxk60  ReadBeforeWriteMsg=warning  WriteAfterWriteMsg=warning  WriteAfterReadMsg=warning  ShowAdditionalParam=off
  Data Store Read : DataStoreRead  DataStoreName=count6  IndexOptions=Index vector (dialog)  Indices=1  OutputSizes=1
  Data Store Read1 : DataStoreRead  DataStoreName=xxk6  IndexOptions=Index vector (dialog)  Indices=1  OutputSizes=1
  Data Store Read10 : DataStoreRead  DataStoreName=vxk60  IndexOptions=Index vector (dialog)  Indices=1  OutputSizes=1
  Data Store Read11 : DataStoreRead  DataStoreName=vyk60  IndexOptions=Index vector (dialog)  Indices=1  OutputSizes=1
  Data Store Read12 : DataStoreRead  DataStoreName=vzk60  IndexOptions=Index vector (dialog)  Indices=1  OutputSizes=1
  Data Store Read2 : DataStoreRead  DataStoreName=xyk6  IndexOptions=Index vector (dialog)  Indices=1  OutputSizes=1
  Data Store Read3 : DataStoreRead  DataStoreName=xzk6  IndexOptions=Index vector (dialog)  Indices=1  OutputSizes=1
  Data Store Read4 : DataStoreRead  DataStoreName=vxk6  IndexOptions=Index vector (dialog)  Indices=1  OutputSizes=1
  Data Store Read5 : DataStoreRead  DataStoreName=vyk6  IndexOptions=Index vector (dialog)  Indices=1  OutputSizes=1
  Data Store Read6 : DataStoreRead  DataStoreName=vzk6  IndexOptions=Index vector (dialog)  Indices=1  OutputSizes=1
  Data Store Read7 : DataStoreRead  DataStoreName=xxk60  IndexOptions=Index vector (dialog)  Indices=1  OutputSizes=1
  Data Store Read8 : DataStoreRead  DataStoreName=xyk60  IndexOptions=Index vector (dialog)  Indices=1  OutputSizes=1
  Data Store Read9 : DataStoreRead  DataStoreName=xzk60  IndexOptions=Index vector (dialog)  Indices=1  OutputSizes=1
  Data Store Write : DataStoreWrite  DataStoreName=count6  IndexOptions=Index vector (dialog)  Indices=1  OutputSizes=1
  Data Store Write1 : DataStoreWrite  DataStoreName=xxk6  IndexOptions=Index vector (dialog)  Indices=1  OutputSizes=1
  Data Store Write10 : DataStoreWrite  DataStoreName=vxk60  IndexOptions=Index vector (dialog)  Indices=1  OutputSizes=1
  Data Store Write11 : DataStoreWrite  DataStoreName=vyk60  IndexOptions=Index vector (dialog)  Indices=1  OutputSizes=1
  Data Store Write12 : DataStoreWrite  DataStoreName=vzk60  IndexOptions=Index vector (dialog)  Indices=1  OutputSizes=1
  Data Store Write2 : DataStoreWrite  DataStoreName=xyk6  IndexOptions=Index vector (dialog)  Indices=1  OutputSizes=1
  Data Store Write3 : DataStoreWrite  DataStoreName=xzk6  IndexOptions=Index vector (dialog)  Indices=1  OutputSizes=1
  Data Store Write4 : DataStoreWrite  DataStoreName=vxk6  IndexOptions=Index vector (dialog)  Indices=1  OutputSizes=1
  Data Store Write5 : DataStoreWrite  DataStoreName=vyk6  IndexOptions=Index vector (dialog)  Indices=1  OutputSizes=1
  Data Store Write6 : DataStoreWrite  DataStoreName=vzk6  IndexOptions=Index vector (dialog)  Indices=1  OutputSizes=1
  Data Store Write7 : DataStoreWrite  DataStoreName=xxk60  IndexOptions=Index vector (dialog)  Indices=1  OutputSizes=1
  Data Store Write8 : DataStoreWrite  DataStoreName=xyk60  IndexOptions=Index vector (dialog)  Indices=1  OutputSizes=1
  Data Store Write9 : DataStoreWrite  DataStoreName=xzk60  IndexOptions=Index vector (dialog)  Indices=1  OutputSizes=1
  Demux1 : Demux  Outputs=12
  Display : Display
  L+B : Subsystem
  MATLAB Function : MATLAB Function  TreatAsAtomicUnit=on
  MATLAB Function2 : MATLAB Function  TreatAsAtomicUnit=on
  MATLAB Function3 : MATLAB Function  TreatAsAtomicUnit=on
  Memory : Memory
  Mux1 : Mux  Inputs=3
  Mux2 : Mux  Inputs=3
  Mux3 : Mux  Inputs=12
  Mux4 : Mux  Inputs=12
  Product : Product
  Product1 : Product
  Subsystem1 : Subsystem
  Subsystem2 : Subsystem
  Subsystem3 : Subsystem
  Subsystem4 : Subsystem
  Subsystem5 : Subsystem
  Subsystem6 : Subsystem
  Subtract : Sum  Inputs=+-
  Switch : Switch  Criteria=u2 > Threshold
  Switch2 : Switch  Criteria=u2 > Threshold
  u6 : Outport
  wires:
  Subsystem1/1(utx) -> Mux2/2
  Subsystem6/1(utx) -> Mux2/1
  Subsystem2/1(utx) -> Mux2/3
  Data Store Read/1 -> Add/2
  Subsystem3/1(ey) -> Mux1/2
  MATLAB Function/1(y) -> Product/1
  Mux2/1 -> MATLAB Function/1(u)
  Product1/1 -> Subtract/1
  Add/1 -> Data Store Write/1, Display/1
  Subsystem5/1(ex) -> Mux1/1
  Subsystem4/1(ez) -> Mux1/3
  Mux1/1 -> MATLAB Function2/1(u)
  MATLAB Function2/1(y) -> Product1/1
  Constant4/1 -> Switch2/1
  Constant/1 -> Product/2
  Constant5/1 -> Switch2/3
  MATLAB Function3/1(y) -> Product1/2
  Switch2/1 -> Add/1  "e1"
  Product/1 -> Subtract/2
  Memory/1 -> u6/1  "node6"
  Bus Selector4/4 -> Subsystem5/4(vx)  "<vx>"
  Bus Selector5/3 -> Subsystem3/3(vyk)  "<vy>"
  Bus Selector5/2 -> Subsystem3/2(xy)  "<xy>"
  Bus Selector4/1 -> Subsystem5/1(xxk)  "<xx>"
  Bus Selector5/4 -> Subsystem3/4(vy)  "<vy>"
  Bus Selector5/1 -> Subsystem3/1(xyk)  "<xy>"
  In19/1 -> Bus Selector1/1, Bus Selector2/1, [state], Bus Selector/1, Bus Selector5/1, Bus Selector4/1, Bus Selector6/1
  Bus Selector4/3 -> Subsystem5/3(vxk)  "<vx>"
  Bus Selector6/2 -> Subsystem4/2(xz)  "<xz>"
  Bus Selector6/3 -> Subsystem4/3(vzk)  "<vz>"
  Bus Selector4/2 -> Subsystem5/2(xx)  "<xx>"
  Bus Selector6/4 -> Subsystem4/4(vz)  "<vz>"
  Bus Selector6/1 -> Subsystem4/1(xzk)  "<xz>"
  Subtract/1 -> Switch/2, Switch2/2
  Demux1/3 -> Data Store Write3/1, Bus Creator3/3  "xz"
  Demux1/12 -> Bus Creator3/12, Data Store Write12/1  "vz0"
  Demux1/9 -> Data Store Write9/1, Bus Creator3/9  "xz0"
  Data Store Read3/1 -> Mux3/3
  Bus Selector7/10 -> Mux4/10  "<vx>"
  Data Store Read2/1 -> Mux3/2
  Mux3/1 -> Switch/3
  Demux1/10 -> Data Store Write10/1, Bus Creator3/10  "vx0"
  Bus Selector7/5 -> Mux4/5  "<vy>"
  Data Store Read6/1 -> Mux3/6
  Data Store Read5/1 -> Mux3/5
  Demux1/5 -> Data Store Write5/1, Bus Creator3/5  "vy"
  Data Store Read1/1 -> Mux3/1
  Demux1/11 -> Data Store Write11/1, Bus Creator3/11  "vy0"
  Demux1/1 -> Data Store Write1/1, Bus Creator3/1  "xx"
  Data Store Read4/1 -> Mux3/4
  [state] -> Bus Selector7/1
  Data Store Read11/1 -> Mux3/11
  Demux1/6 -> Data Store Write6/1, Bus Creator3/6  "vz"
  Bus Selector7/2 -> Mux4/2  "<xy>"
  Bus Selector7/1 -> Mux4/1  "<xx>"
  Bus Selector7/8 -> Mux4/8  "<xy>"
  Data Store Read10/1 -> Mux3/10
  Bus Selector7/4 -> Mux4/4  "<vx>"
  Mux4/1 -> Switch/1
  Data Store Read12/1 -> Mux3/12
  Bus Creator3/1 -> Memory/1
  Bus Selector7/7 -> Mux4/7  "<xx>"
  Bus Selector7/6 -> Mux4/6  "<vz>"
  Demux1/2 -> Data Store Write2/1, Bus Creator3/2  "xy"
  Demux1/4 -> Data Store Write4/1, Bus Creator3/4  "vx"
  Data Store Read9/1 -> Mux3/9
  Bus Selector7/11 -> Mux4/11  "<vy>"
  Bus Selector7/9 -> Mux4/9  "<xz>"
  Demux1/8 -> Data Store Write8/1, Bus Creator3/8  "xy0"
  Demux1/7 -> Data Store Write7/1, Bus Creator3/7  "xx0"
  Bus Selector7/3 -> Mux4/3  "<xz>"
  Data Store Read7/1 -> Mux3/7
  Data Store Read8/1 -> Mux3/8
  Switch/1 -> Demux1/1
  Bus Selector7/12 -> Mux4/12  "<vz>"
  Bus Selector/2 -> Subsystem6/2(xx0)  "<xx0>"
  Bus Selector1/4 -> Subsystem1/4(xx2)  "<xy>"
  Bus Selector/8 -> Subsystem6/8(vx2)  "<vx>"
  Bus Selector1/5 -> Subsystem1/5(vx6)  "<vy>"
  Bus Selector/6 -> Subsystem6/6(vx0)  "<vx0>"
  Bus Selector1/7 -> Subsystem1/7(vx1)  "<vy>"
  Bus Selector1/2 -> Subsystem1/2(xx0)  "<xy0>"
  Bus Selector1/1 -> Subsystem1/1(xx6)  "<xy>"
  Bus Selector2/1 -> Subsystem2/1(xx6)  "<xz>"
  Bus Selector2/6 -> Subsystem2/6(vx0)  "<vz0>"
  Bus Selector2/5 -> Subsystem2/5(vx6)  "<vz>"
  Bus Selector/5 -> Subsystem6/5(vx6)  "<vx>"
  Bus Selector/7 -> Subsystem6/7(vx1)  "<vx>"
  Bus Selector1/8 -> Subsystem1/8(vx2)  "<vy>"
  Bus Selector2/2 -> Subsystem2/2(xx0)  "<xz0>"
  Bus Selector2/4 -> Subsystem2/4(xx2)  "<xz>"
  Bus Selector/4 -> Subsystem6/4(xx2)  "<xx>"
  Bus Selector/1 -> Subsystem6/1(xx6)  "<xx>"
  Bus Selector1/6 -> Subsystem1/6(vx0)  "<vy0>"
  Bus Selector1/3 -> Subsystem1/3(xx1)  "<xy>"
  Bus Selector/3 -> Subsystem6/3(xx1)  "<xx>"
  Bus Selector2/3 -> Subsystem2/3(xx1)  "<xz>"
  Bus Selector2/7 -> Subsystem2/7(vx1)  "<vz>"
  Bus Selector2/8 -> Subsystem2/8(vx2)  "<vz>"
  L+B/1(u) -> MATLAB Function3/1(u)

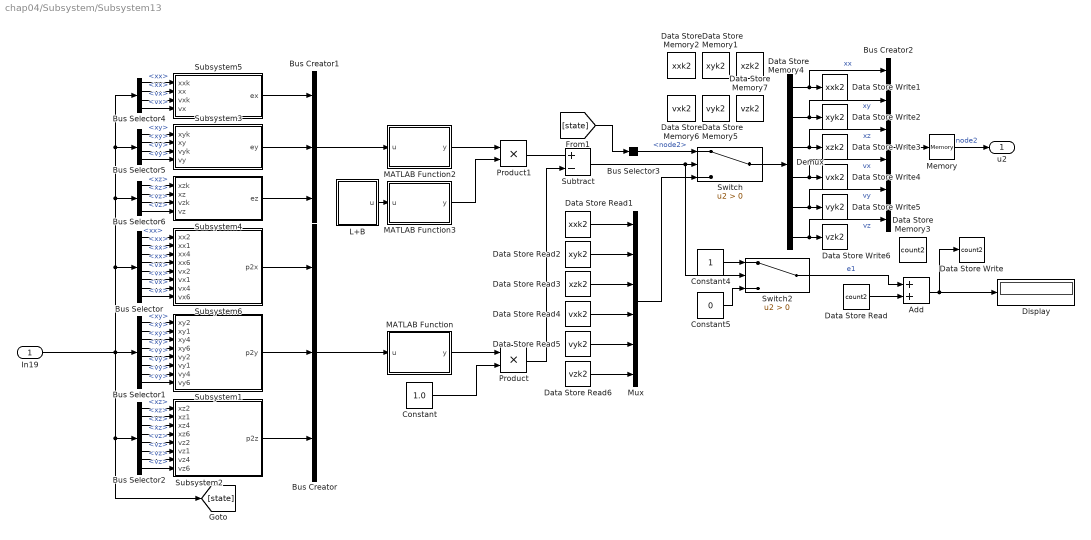
== system chap04/Subsystem/Subsystem13 ==
  In19 : Inport
  Add : Sum
  Bus Creator : BusCreator  Inputs=3
  Bus Creator1 : BusCreator  Inputs=3
  Bus Creator2 : BusCreator  Inputs=6
  Bus Selector : BusSelector  OutputSignals=state(tk).node2.xx,state(tk).node1.xx,state(tk).node4.xx,state(tk).node6.xx,state(tk).node2.vx,state(tk).node1.vx,state(tk).node4.vx,state(tk).node6.vx
  Bus Selector1 : BusSelector  OutputSignals=state(tk).node2.xy,state(tk).node1.xy,state(tk).node4.xy,state(tk).node6.xy,state(tk).node2.vy,state(tk).node1.vy,state(tk).node4.vy,state(tk).node6.vy
  Bus Selector2 : BusSelector  OutputSignals=state(tk).node2.xz,state(tk).node1.xz,state(tk).node4.xz,state(tk).node6.xz,state(tk).node2.vz,state(tk).node1.vz,state(tk).node4.vz,state(tk).node6.vz
  Bus Selector3 : BusSelector  OutputSignals=state(t).node2
  Bus Selector4 : BusSelector  OutputSignals=state(tk).node2.xx,state(t).node2.xx,state(tk).node2.vx,state(t).node2.vx
  Bus Selector5 : BusSelector  OutputSignals=state(tk).node2.xy,state(t).node2.xy,state(tk).node2.vy,state(t).node2.vy
  Bus Selector6 : BusSelector  OutputSignals=state(tk).node2.xz,state(t).node2.xz,state(tk).node2.vz,state(t).node2.vz
  Constant : Constant  Value=1.0
  Constant4 : Constant
  Constant5 : Constant  Value=0
  Data Store Memory1 : DataStoreMemory  DataStoreName=xyk2  ReadBeforeWriteMsg=warning  WriteAfterWriteMsg=warning  WriteAfterReadMsg=warning  ShowAdditionalParam=off
  Data Store Memory2 : DataStoreMemory  DataStoreName=xxk2  ReadBeforeWriteMsg=warning  WriteAfterWriteMsg=warning  WriteAfterReadMsg=warning  ShowAdditionalParam=off
  Data Store Memory3 : DataStoreMemory  DataStoreName=count2  ReadBeforeWriteMsg=warning  WriteAfterWriteMsg=warning  WriteAfterReadMsg=warning  ShowAdditionalParam=off
  Data Store Memory4 : DataStoreMemory  DataStoreName=xzk2  ReadBeforeWriteMsg=warning  WriteAfterWriteMsg=warning  WriteAfterReadMsg=warning  ShowAdditionalParam=off
  Data Store Memory5 : DataStoreMemory  DataStoreName=vyk2  ReadBeforeWriteMsg=warning  WriteAfterWriteMsg=warning  WriteAfterReadMsg=warning  ShowAdditionalParam=off
  Data Store Memory6 : DataStoreMemory  DataStoreName=vxk2  ReadBeforeWriteMsg=warning  WriteAfterWriteMsg=warning  WriteAfterReadMsg=warning  ShowAdditionalParam=off
  Data Store Memory7 : DataStoreMemory  DataStoreName=vzk2  ReadBeforeWriteMsg=warning  WriteAfterWriteMsg=warning  WriteAfterReadMsg=warning  ShowAdditionalParam=off
  Data Store Read : DataStoreRead  DataStoreName=count2  IndexOptions=Index vector (dialog)  Indices=1  OutputSizes=1
  Data Store Read1 : DataStoreRead  DataStoreName=xxk2  IndexOptions=Index vector (dialog)  Indices=1  OutputSizes=1
  Data Store Read2 : DataStoreRead  DataStoreName=xyk2  IndexOptions=Index vector (dialog)  Indices=1  OutputSizes=1
  Data Store Read3 : DataStoreRead  DataStoreName=xzk2  IndexOptions=Index vector (dialog)  Indices=1  OutputSizes=1
  Data Store Read4 : DataStoreRead  DataStoreName=vxk2  IndexOptions=Index vector (dialog)  Indices=1  OutputSizes=1
  Data Store Read5 : DataStoreRead  DataStoreName=vyk2  IndexOptions=Index vector (dialog)  Indices=1  OutputSizes=1
  Data Store Read6 : DataStoreRead  DataStoreName=vzk2  IndexOptions=Index vector (dialog)  Indices=1  OutputSizes=1
  Data Store Write : DataStoreWrite  DataStoreName=count2  IndexOptions=Index vector (dialog)  Indices=1  OutputSizes=1
  Data Store Write1 : DataStoreWrite  DataStoreName=xxk2  IndexOptions=Index vector (dialog)  Indices=1  OutputSizes=1
  Data Store Write2 : DataStoreWrite  DataStoreName=xyk2  IndexOptions=Index vector (dialog)  Indices=1  OutputSizes=1
  Data Store Write3 : DataStoreWrite  DataStoreName=xzk2  IndexOptions=Index vector (dialog)  Indices=1  OutputSizes=1
  Data Store Write4 : DataStoreWrite  DataStoreName=vxk2  IndexOptions=Index vector (dialog)  Indices=1  OutputSizes=1
  Data Store Write5 : DataStoreWrite  DataStoreName=vyk2  IndexOptions=Index vector (dialog)  Indices=1  OutputSizes=1
  Data Store Write6 : DataStoreWrite  DataStoreName=vzk2  IndexOptions=Index vector (dialog)  Indices=1  OutputSizes=1
  Demux : Demux  Outputs=6
  Display : Display
  L+B : Subsystem
  MATLAB Function : MATLAB Function  TreatAsAtomicUnit=on
  MATLAB Function2 : MATLAB Function  TreatAsAtomicUnit=on
  MATLAB Function3 : MATLAB Function  TreatAsAtomicUnit=on
  Memory : Memory
  Mux : Mux  Inputs=6
  Product : Product
  Product1 : Product
  Subsystem1 : Subsystem
  Subsystem2 : Subsystem
  Subsystem3 : Subsystem
  Subsystem4 : Subsystem
  Subsystem5 : Subsystem
  Subsystem6 : Subsystem
  Subtract : Sum  Inputs=+-
  Switch : Switch  Criteria=u2 > Threshold
  Switch2 : Switch  Criteria=u2 > Threshold
  u2 : Outport
  wires:
  Bus Selector2/8 -> Subsystem2/8(vz6)  "<vz>"
  Bus Selector2/7 -> Subsystem2/7(vz4)  "<vz>"
  Bus Selector2/6 -> Subsystem2/6(vz1)  "<vz>"
  Bus Selector2/5 -> Subsystem2/5(vz2)  "<vz>"
  Bus Selector2/4 -> Subsystem2/4(xz6)  "<xz>"
  Bus Selector2/3 -> Subsystem2/3(xz4)  "<xz>"
  Bus Selector2/2 -> Subsystem2/2(xz1)  "<xz>"
  Bus Selector2/1 -> Subsystem2/1(xz2)  "<xz>"
  Bus Selector1/8 -> Subsystem1/8(vy6)  "<vy>"
  Bus Selector1/7 -> Subsystem1/7(vy4)  "<vy>"
  Bus Selector1/6 -> Subsystem1/6(vy1)  "<vy>"
  Bus Selector1/5 -> Subsystem1/5(vy2)  "<vy>"
  Bus Selector1/4 -> Subsystem1/4(xy6)  "<xy>"
  Bus Selector1/3 -> Subsystem1/3(xy4)  "<xy>"
  Bus Selector1/2 -> Subsystem1/2(xy1)  "<xy>"
  Bus Selector1/1 -> Subsystem1/1(xy2)  "<xy>"
  Bus Selector/8 -> Subsystem6/8(vx6)  "<vx>"
  Bus Selector/7 -> Subsystem6/7(vx4)  "<vx>"
  Bus Selector/6 -> Subsystem6/6(vx1)  "<vx>"
  Bus Selector/5 -> Subsystem6/5(vx2)  "<vx>"
  Bus Selector/4 -> Subsystem6/4(xx6)  "<xx>"
  Bus Selector/3 -> Subsystem6/3(xx4)  "<xx>"
  Bus Selector/2 -> Subsystem6/2(xx1)  "<xx>"
  Bus Selector/1 -> Subsystem6/1(xx2)  "<xx>"
  Subsystem2/1(p2z) -> Bus Creator/3
  Subsystem6/1(p2x) -> Bus Creator/1
  Subsystem1/1(p2y) -> Bus Creator/2
  Subsystem3/1(ey) -> Bus Creator1/2
  Subsystem4/1(ez) -> Bus Creator1/3
  MATLAB Function3/1(y) -> Product1/2
  Constant/1 -> Product/2
  MATLAB Function2/1(y) -> Product1/1
  MATLAB Function/1(y) -> Product/1
  Subsystem5/1(ex) -> Bus Creator1/1
  Bus Creator1/1 -> MATLAB Function2/1(u)
  Bus Creator/1 -> MATLAB Function/1(u)
  Data Store Read5/1 -> Mux/5
  Data Store Read/1 -> Add/2
  Product1/1 -> Subtract/1
  Add/1 -> Data Store Write/1, Display/1
  Mux/1 -> Switch/3
  Constant4/1 -> Switch2/1
  Data Store Read3/1 -> Mux/3
  Data Store Read1/1 -> Mux/1
  Bus Selector3/1 -> Switch/1  "<node2>"
  Constant5/1 -> Switch2/3
  Switch2/1 -> Add/1  "e1"
  Data Store Read6/1 -> Mux/6
  Switch/1 -> Demux/1
  Data Store Read2/1 -> Mux/2
  Data Store Read4/1 -> Mux/4
  Product/1 -> Subtract/2
  [state] -> Bus Selector3/1
  Demux/2 -> Bus Creator2/2, Data Store Write2/1  "xy"
  Demux/1 -> Bus Creator2/1, Data Store Write1/1  "xx"
  Demux/5 -> Bus Creator2/5, Data Store Write5/1  "vy"
  Demux/6 -> Bus Creator2/6, Data Store Write6/1  "vz"
  Demux/3 -> Bus Creator2/3, Data Store Write3/1  "xz"
  Memory/1 -> u2/1  "node2"
  Demux/4 -> Bus Creator2/4, Data Store Write4/1  "vx"
  In19/1 -> [state], Bus Selector2/1, Bus Selector6/1, Bus Selector5/1, Bus Selector4/1, Bus Selector/1, Bus Selector1/1
  Bus Selector4/1 -> Subsystem5/1(xxk)  "<xx>"
  Bus Selector4/2 -> Subsystem5/2(xx)  "<xx>"
  Bus Selector4/3 -> Subsystem5/3(vxk)  "<vx>"
  Bus Selector4/4 -> Subsystem5/4(vx)  "<vx>"
  Bus Selector5/1 -> Subsystem3/1(xyk)  "<xy>"
  Bus Selector5/2 -> Subsystem3/2(xy)  "<xy>"
  Bus Selector5/3 -> Subsystem3/3(vyk)  "<vy>"
  Bus Selector5/4 -> Subsystem3/4(vy)  "<vy>"
  Bus Selector6/1 -> Subsystem4/1(xzk)  "<xz>"
  Bus Selector6/2 -> Subsystem4/2(xz)  "<xz>"
  Bus Selector6/3 -> Subsystem4/3(vzk)  "<vz>"
  Bus Selector6/4 -> Subsystem4/4(vz)  "<vz>"
  Bus Creator2/1 -> Memory/1
  Subtract/1 -> Switch/2, Switch2/2
  L+B/1(u) -> MATLAB Function3/1(u)
